simulink model "TEG_MPPT_PO_Benchmark"  (R2021b)
settings: Solver=ode45  StartTime=0.0  StopTime=0.1  RelTol=1e-3  EnableMultiTasking=on
values from neighbouring files (symbols this model uses):
  delta_T = Th - Tc    (= 380)    [TEG_BenchmarkStart.m]
  m = 1    [TEG_BenchmarkStart.m]
  RL = (Vm^2)/Wm    (= 7.2)    [TEG_BenchmarkStart.m]
  Tc = Tc + 273.15    (= 293.15)    [TEG_BenchmarkStart.m]
  Th = Th + 273.15    (= 673.15)    [TEG_BenchmarkStart.m]
  Vm = 1.2    [TEG_BenchmarkStart.m]
  Wm = 0.2    [TEG_BenchmarkStart.m]
undefined symbols (not defined in the file or in its folder): Ion, Lithium
libraries: spsSeriesRLCBranchLib x3, spsCurrentMeasurementLib x2, simulink x2, spsPWMGeneratorDCDCLib x2, spsVoltageMeasurementLib x2, spsBatteryLib x1, spsControlledVoltageSourceLib x1, spsDiodeLib x1, spsMeanLib x1, spsMosfetLib x1, spspowerguiLib x1
settings Model: Creator=nitukeee  LastModifiedBy=romem
settings SolverCC: ZeroCrossAlgorithm=Adaptive  AlgebraicLoopSolver=TrustRegion
settings DataIOCC: LimitDataPoints=on  SaveFormat=Array  ReturnWorkspaceOutputs=off
settings OptimizationCC: LifeSpan=inf
settings DebuggingCC: SolverPrmCheckMsg=warning  SFUnexpectedBacktrackingDiag=warning  SFNoUnconditionalDefaultTransitionDiag=warning  SFExecutionAtInitializationDiag=none  SFMachineParentedDataDiag=warning  ArithmeticOperatorsInVariantConditions=warning
settings HardwareCC: ProdBitPerPointer=32  ProdBitPerSizeT=32  ProdBitPerPtrDiffT=32  ProdLargestAtomicFloat=None  ProdIntDivRoundTo=Undefined  ProdEndianess=Unspecified  ProdWordSize=32  ProdHWDeviceType=32-bit Generic
settings ModelReferenceCC: PropagateSignalLabelsOutOfModel=off
settings SFSimCC: SimUseLocalCustomCode=off  CustomCodeUndefinedFunction=UseInterfaceOnly
settings RTWCC: RTWUseLocalCustomCode=off
settings CodeAppCC: StateflowObjectComments=on
settings GRTTargetCC: TargetLangStandard=C89/C90 (ANSI)
settings ConfigComp: CovMetricSettings=dw  CovSaveCumulativeToWorkspaceVar=on  CovSaveSingleToWorkspaceVar=on  CovExternalEMLEnable=off  CovSFcnEnable=off
settings SimscapeCC: SimscapeNormalizeSystem=off

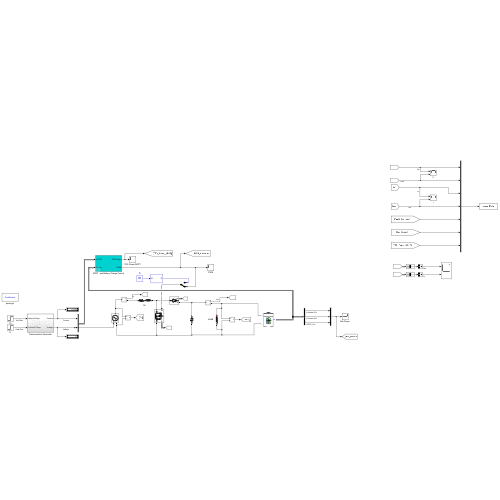
[thumbnail: Simulink's stored preview of the top-level diagram]
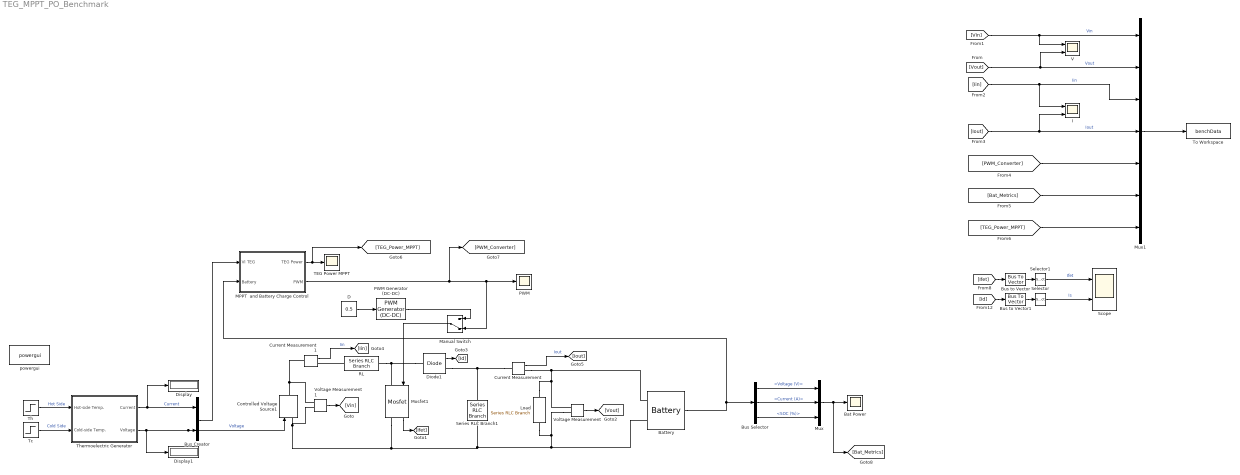
== system TEG_MPPT_PO_Benchmark ==
  Bat Power : Scope
  Battery : spsBatteryLib/Battery  BatType=Lithium-Ion  ShowTempParam=off  ThermalPreset="3.7V  4.4Ah"  ShowAgeParam=off  NomV=3.4  NomQ=4.4  SOC=10  Batt_Tr=5  PresetModel=off  MaxQ=4.5  MinV=2.55  FullV=4.125  Dis_rate=0.9  R=0.00818  Normal_OP=4  expZone="[4         0.5]"  current=[6.5 13 32.5]  Units=Time  Tci=20  NomT=20  T2=-30  MaxQ2=3.8  FullV2=3.38  Normal_OP2=2.75  expZone2="[3.25         0.5]"  Rca=0.06  ti=1000  Dp=0  Neq0=0  Tsim=1e6  Ta1=25  Qeol=5.4*0.9  Reol=0.013333*1.2  Char_age=[2.3478, 3]  Dis_age=[2.3478, 10]  N1=1500  N2=10500  N3=1000  N4=1400  Ta2=45  N5=950
  Bus Creator : BusCreator  Inputs=2
  Bus Selector : BusSelector  OutputSignals=Voltage (V),Current (A),SOC (%)
  Bus to Vector : BusToVector
  Bus to Vector1 : BusToVector
  Controlled Voltage Source1 : spsControlledVoltageSourceLib/Controlled Voltage Source  Initialize=on  Source_Type=DC  Amplitude=0  Phase=0  Frequency=0  Measurements=None
  Current Measurement : spsCurrentMeasurementLib/Current Measurement  PhasorSimulation=off  OutputType=Complex  PSBequivalent=0
  Current Measurement1 : spsCurrentMeasurementLib/Current Measurement  PhasorSimulation=off  OutputType=Complex  PSBequivalent=0
  D : Constant  Value=0.5
  Diode1 : spsDiodeLib/Diode  Ron=1e-3  Lon=0  Vf=0  IC=0  UseSnubber=off  Rs=inf  Cs=inf  Measurements=on
  Display : Display
  Display1 : Display
  I : Scope  NumInputPorts=2
  Load : spsSeriesRLCBranchLib/Series RLC Branch  LConnTagsString=__new0  RConnTagsString=__new0  BranchType=R  Resistance=100  Inductance=200e-6  SetiL0=off  InitialCurrent=0  Capacitance=400e-6  Setx0=off  InitialVoltage=0  Measurements=None
  MPPT  and Battery Charge Control : Subsystem  mask(MPPT Solar Charge Controller Block){dD=1e-6, BattCV=3.7, Fsw=20e3}
      mask prompts: dD "MPPT Duty Cycle (delta) Step Size"; BattCV "Battery Charging Constant Voltage (V)"; Fsw "PWM Switching frequency (Hz):"
      mask help:
      | MPPT Solar Charge Controller Block
      | Developed by Rodney Tan (PhD)
      | Version 1.00 Oct 2019
      |
      | This block perform solar photovoltaic Maximum Power Point Tracking based on Perturbation & Observation algorithm and charge lead acid battery using three stage charging algorithm.
      mask Help:
      | <b><u>Block Setting</u></b>
      | 
      | <b>MPPT Duty Cycle Step Size</b>
      | Specify the MPPT duty cycle (delta) step size. Default value is 1e-5.
      | 
      | <b>Battery Charging Constant Voltage (V)</b>
      | Specify the battery charging constant voltage for absorption stage.
      | 
      | <b>PWM Switching Frequency (Hz)</b>
      | Specify the PWM switching frequency in Hz.
      mask TypeOptions Fsw:
      | PWM Generator
      | (DC-DC)/Fsw
  Manual Switch : ManualSwitch  CurrentSetting=0
  Mosfet1 : spsMosfetLib/Mosfet  Ron=1e-3  Lon=0  Rd=1e-3  Vfd=0  IC=0  Rs=inf  Cs=inf  Measurements=on
  Mux : Mux  Inputs=3
  Mux1 : Mux  Inputs=7
  PWM : Scope
  PWM Generator (DC-DC) : spsPWMGeneratorDCDCLib/PWM Generator (DC-DC)  Fsw=20e3  Ts=0
  RL : spsSeriesRLCBranchLib/Series RLC Branch  LConnTagsString=__new0  RConnTagsString=__new0  BranchType=RL  Resistance=1e-3  Inductance=250e-6  SetiL0=off  InitialCurrent=0  Capacitance=1e-6  Setx0=off  InitialVoltage=0  Measurements=None
  Scope : Scope  NumInputPorts=2
  Selector : Selector  InputPortWidth=2  IndexOptions=Index vector (dialog)  Indices=1  OutputSizes=1
  Selector1 : Selector  InputPortWidth=2  IndexOptions=Index vector (dialog)  Indices=1  OutputSizes=1
  Series RLC Branch1 : spsSeriesRLCBranchLib/Series RLC Branch  LConnTagsString=__new0  RConnTagsString=__new0  BranchType=C  Resistance=1e-4  Inductance=200e-6  SetiL0=off  InitialCurrent=0  Capacitance=200e-6  Setx0=off  InitialVoltage=40  Measurements=None
  TEG Power MPPT : Scope
  Tc : Step  Time=0  After=Tc  SampleTime=0
  Th : Step  Time=0  After=Th  SampleTime=0
  Thermoelectric Generator : Subsystem
  To Workspace : ToWorkspace  VariableName=benchData  SaveFormat=Timeseries  SampleTime=-1
  V : Scope  NumInputPorts=2
  Voltage Measurement : spsVoltageMeasurementLib/Voltage Measurement  PhasorSimulation=off  OutputType=Complex  PSBequivalent=0
  Voltage Measurement1 : spsVoltageMeasurementLib/Voltage Measurement  PhasorSimulation=off  OutputType=Complex  PSBequivalent=0
  powergui : spspowerguiLib/powergui  Priority=1  SimulationMode=Continuous  SampleTime=50e-6  frequency=60  Iterations=50  frequencyindice=0  Pbase=100e6  ErrMax=1e-4  UnitsV=kV  UnitsW=MW  buscounter=0  FunctionMessages=off  echomessages=off  EnableUseOfTLC=off  CurrentSourceSwitches=off  DisableSnubberDevices=off  DisableRonSwitches=off  DisableVfSwitches=off  DisplayEquations=off  AutomaticDiscreteSolvers=off  SolverType=Tustin/Backward Euler (TBE)  Interpol=off  ExternalGateDelay=off  methode=off  Ts=100  x0status=blocks  SPID=on  SwTol=0  HookPort=off  NonlinearTolerance=1e-4  nMaxIteration=100  ContinueOnMaxIteration=off  RestoreLinks=warning  ResistiveCurrentMeasurement=off  Frange=[0:2:500]  Ylog=off  Xlog=on  ShowGrid=off  save=off  variable=ZData  structure=0  ZoomFFT=off  StartTime=0.0  cycles=1  DisplayStyle=1  fundamental=60  FreqAxis=off  MaxFrequency=1000  frequencyindicesteady=1  RmsSteady=1  display=off
  wires:
  [Id] -> Bus to Vector1/1
  Diode1/1 -> [Id]
  Selector/1 -> Scope/2  "Is"
  Bus Selector/2 -> Mux/2  "<Current (A)>"
  [TEG_Power_MPPT] -> Mux1/7
  Bus Selector/1 -> Mux/1  "<Voltage (V)>"
  [Bat_Metrics] -> Mux1/6
  [Ifet] -> Bus to Vector/1
  [PWM_Converter] -> Mux1/5
  Bus to Vector1/1 -> Selector/1
  [Iin] -> Mux1/3, I/1  "Iin"
  Th/1 -> Thermoelectric Generator/1(Hot-side Temp.)  "Hot Side"
  Thermoelectric Generator/1(Current) -> Display/1, Bus Creator/1  "Current"
  Tc/1 -> Thermoelectric Generator/2(Cold-side Temp.)  "Cold Side"
  Battery/1 -> MPPT  and Battery Charge Control/2(Battery), Bus Selector/1
  Mux1/1 -> To Workspace/1
  Manual Switch/1 -> Mosfet1/1
  [Iout] -> I/2, Mux1/4  "Iout"
  Mux/1 -> [Bat_Metrics], Bat Power/1
  PWM Generator (DC-DC)/1 -> Manual Switch/1
  Bus Creator/1 -> MPPT  and Battery Charge Control/1(VI TEG)
  MPPT  and Battery Charge Control/2(PWM) -> [PWM_Converter], PWM/1, Manual Switch/2
  [Vin] -> V/1, Mux1/1  "Vin"
  Thermoelectric Generator/2(Voltage) -> Display1/1, Controlled Voltage Source1/1, Bus Creator/2  "Voltage"
  Current Measurement/1 -> [Iout]  "Iout"
  Voltage Measurement1/1 -> [Vin]
  Current Measurement1/1 -> [Iin]  "Iin"
  Mosfet1/1 -> [Ifet]
  Bus to Vector/1 -> Selector1/1
  D/1 -> PWM Generator (DC-DC)/1
  [Vout] -> V/2, Mux1/2  "Vout"
  MPPT  and Battery Charge Control/1(TEG Power) -> [TEG_Power_MPPT], TEG Power MPPT/1
  Bus Selector/3 -> Mux/3  "<SOC (%)>"
  Voltage Measurement/1 -> [Vout]
  Selector1/1 -> Scope/1  "Ifet"
  connections:
  Load/LConn1 -- Voltage Measurement/LConn1 -- Battery/LConn1 -- Current Measurement/RConn1
  Current Measurement1/LConn1 -- Voltage Measurement1/LConn1 -- Controlled Voltage Source1/RConn1
  Voltage Measurement/LConn2 -- Load/RConn1 -- Battery/LConn2 -- Voltage Measurement1/LConn2 -- Controlled Voltage Source1/LConn1 -- Mosfet1/RConn1 -- Series RLC Branch1/RConn1
  Current Measurement/LConn1 -- Series RLC Branch1/LConn1 -- Diode1/RConn1
  Diode1/LConn1 -- RL/RConn1 -- Mosfet1/LConn1
  RL/LConn1 -- Current Measurement1/RConn1

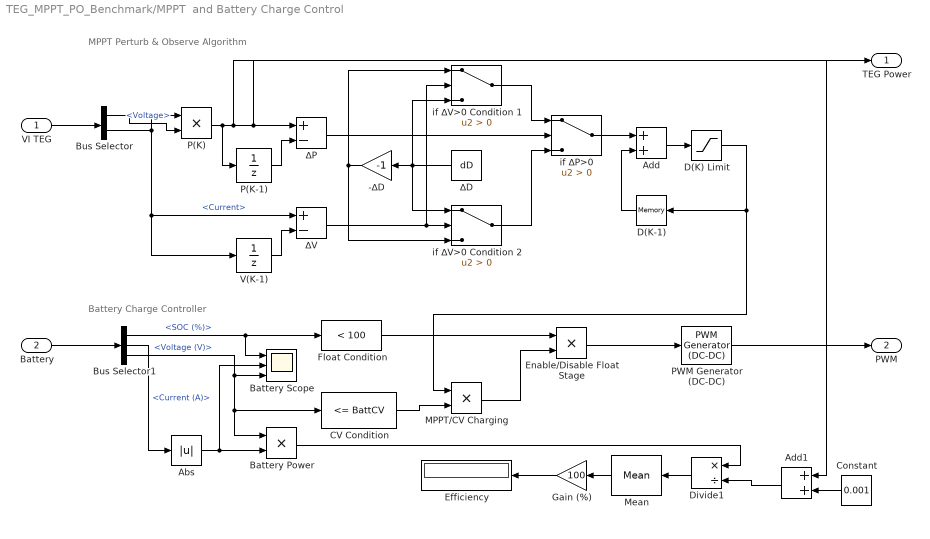
== system TEG_MPPT_PO_Benchmark/MPPT  and Battery Charge Control ==
  note: Battery Charge Controller
  note: MPPT Perturb & Observe Algorithm
  VI TEG : Inport
  Battery : Inport  Port=2
  -∆D : Gain  Gain=-1
  Abs : Abs
  Add : Sum
  Add1 : Sum
  Battery Power : Product
  Battery Scope : Scope  NumInputPorts=3
  Bus Selector : BusSelector  OutputSignals=Voltage,Current
  Bus Selector1 : BusSelector  OutputSignals=SOC (%),Current (A),Voltage (V)
  CV Condition : simulink/Logic and Bit Operations/Compare To Constant  relop=<=  const=BattCV  OutDataTypeStr=boolean
  Constant : Constant  Value=0.001
  D(K) Limit : Saturate  UpperLimit=0.6  LowerLimit=0.4
  D(K-1) : Memory  InitialCondition=0.5  InheritSampleTime=on  LinearizeMemory=on  LinearizeAsDelay=on
  Divide1 : Product  Inputs=*/
  Efficiency : Display
  Enable/Disable Float Stage : Product
  Float Condition : simulink/Logic and Bit Operations/Compare To Constant  relop=<  const=100  OutDataTypeStr=boolean
  Gain (%) : Gain  Gain=100
  MPPT/CV Charging : Product
  Mean : spsMeanLib/Mean  Freq=1  Vinit=0  Ts=0
      link override Model/integrator: InitialCondition=0
  P(K) : Product
  P(K-1) : UnitDelay  SampleTime=-1  HasFrameUpgradeWarning=on
  PWM Generator (DC-DC) : spsPWMGeneratorDCDCLib/PWM Generator (DC-DC)  Fsw=Fsw  Ts=0
  V(K-1) : UnitDelay  SampleTime=-1  HasFrameUpgradeWarning=on
  if ∆P>0 : Switch  Criteria=u2 > Threshold
  if ∆V>0 Condition 1 : Switch  Criteria=u2 > Threshold
  if ∆V>0 Condition 2 : Switch  Criteria=u2 > Threshold
  ∆D : Constant  Value=dD
  ∆P : Sum  Inputs=+-
  ∆V : Sum  Inputs=+-
  TEG Power : Outport  VectorParamsAs1DForOutWhenUnconnected=off
  PWM : Outport  Port=2  VectorParamsAs1DForOutWhenUnconnected=off
  wires:
  P(K)/1 -> TEG Power/1, ∆P/1, Add1/1, P(K-1)/1
  if ∆V>0 Condition 1/1 -> if ∆P>0/1
  ∆P/1 -> if ∆P>0/2
  P(K-1)/1 -> ∆P/2
  V(K-1)/1 -> ∆V/2
  ∆V/1 -> if ∆V>0 Condition 2/2, if ∆V>0 Condition 1/2
  Add/1 -> D(K) Limit/1
  if ∆V>0 Condition 2/1 -> if ∆P>0/3
  D(K-1)/1 -> Add/2
  ∆D/1 -> if ∆V>0 Condition 2/1, -∆D/1, if ∆V>0 Condition 1/3
  -∆D/1 -> if ∆V>0 Condition 2/3, if ∆V>0 Condition 1/1
  PWM Generator (DC-DC)/1 -> PWM/1
  Enable/Disable Float Stage/1 -> PWM Generator (DC-DC)/1
  Float Condition/1 -> Enable/Disable Float Stage/1
  CV Condition/1 -> MPPT/CV Charging/2
  Bus Selector1/3 -> Battery Scope/3, CV Condition/1, Battery Power/1  "<Voltage (V)>"
  Bus Selector1/1 -> Float Condition/1, Battery Scope/1  "<SOC (%)>"
  MPPT/CV Charging/1 -> Enable/Disable Float Stage/2
  Bus Selector1/2 -> Abs/1  "<Current (A)>"
  Divide1/1 -> Mean/1
  Mean/1 -> Gain (%)/1
  Abs/1 -> Battery Scope/2, Battery Power/2
  Bus Selector/1 -> P(K)/2  "<Voltage>"
  Battery Power/1 -> Divide1/1
  Bus Selector/2 -> P(K)/1, ∆V/1, V(K-1)/1  "<Current>"
  VI TEG/1 -> Bus Selector/1
  if ∆P>0/1 -> Add/1
  D(K) Limit/1 -> D(K-1)/1, MPPT/CV Charging/1
  Gain (%)/1 -> Efficiency/1
  Constant/1 -> Add1/2
  Add1/1 -> Divide1/2
  Battery/1 -> Bus Selector1/1

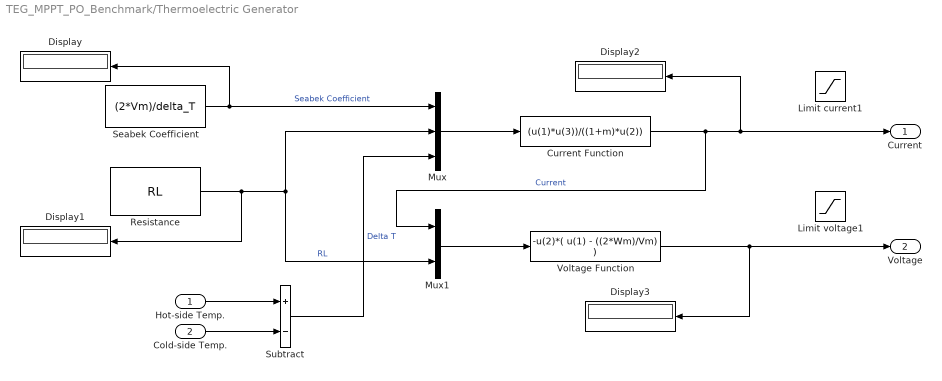
== system TEG_MPPT_PO_Benchmark/Thermoelectric Generator ==
  Hot-side Temp. : Inport
  Cold-side Temp. : Inport  Port=2
  Current Function : Fcn  Expr=(u(1)*u(3))/((1+m)*u(2))
  Display{,1..3} (4 alike) : Display
  Limit current1 : Saturate  UpperLimit=0.170  LowerLimit=0
  Limit voltage1 : Saturate  UpperLimit=1.2  LowerLimit=0
  Mux : Mux  Inputs=3
  Mux1 : Mux  Inputs=2
  Resistance : Constant  Value=RL
  Seabek Coefficient : Constant  Value=(2*Vm)/delta_T
  Subtract : Sum  Inputs=+-
  Voltage Function : Fcn  Expr=-u(2)*( u(1) - ((2*Wm)/Vm) )
  Current : Outport  VectorParamsAs1DForOutWhenUnconnected=off
  Voltage : Outport  Port=2  VectorParamsAs1DForOutWhenUnconnected=off
  wires:
  Hot-side Temp./1 -> Subtract/1
  Cold-side Temp./1 -> Subtract/2
  Current Function/1 -> Display2/1, Current/1, Mux1/1  "Current"
  Mux1/1 -> Voltage Function/1
  Resistance/1 -> Display1/1, Mux1/2, Mux/2  "RL"
  Seabek Coefficient/1 -> Mux/1, Display/1  "Seabek Coefficient"
  Subtract/1 -> Mux/3  "Delta T"
  Mux/1 -> Current Function/1
  Voltage Function/1 -> Display3/1, Voltage/1
